simulink model "MALIBIRAN_MARKVDE_SIMULINK_NO1"  (R2024a)
settings: Solver=VariableStepAuto  StartTime=0.0  StopTime=20  RelTol=1e-3
settings Model: Creator=ninabinay  LastModifiedBy=Doren
settings RTWCC: GPUComputeCapability=3.5

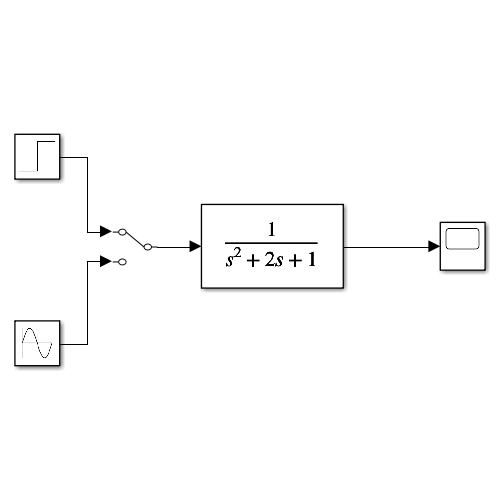
[thumbnail: Simulink's stored preview of the top-level diagram]
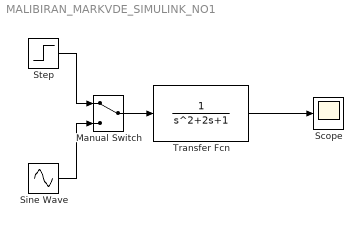
== system MALIBIRAN_MARKVDE_SIMULINK_NO1 ==
  Manual Switch : ManualSwitch
  Scope : Scope
  Sine Wave : Sin  SampleTime=0
  Step : Step  Time=0  SampleTime=0
  Transfer Fcn : TransferFcn
  wires:
  Transfer Fcn/1 -> Scope/1
  Manual Switch/1 -> Transfer Fcn/1
  Sine Wave/1 -> Manual Switch/2
  Step/1 -> Manual Switch/1
